simulink model "car_speed_control_simulation2"  (R2024b)
settings: Solver=VariableStepAuto  StartTime=0.0  StopTime=500  RelTol=1e-3
libraries: simulink_extras x2
settings Model: Creator=USER  LastModifiedBy=USER

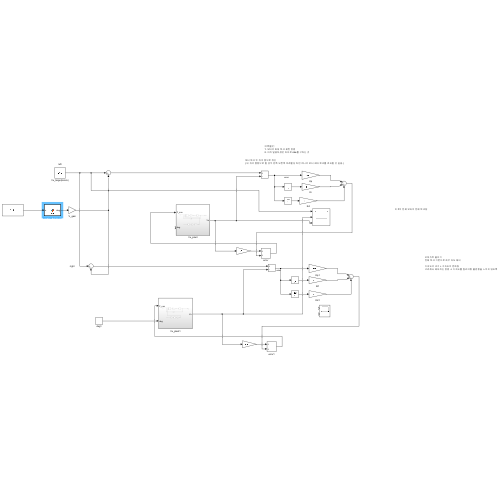
[thumbnail: Simulink's stored preview of the top-level diagram]
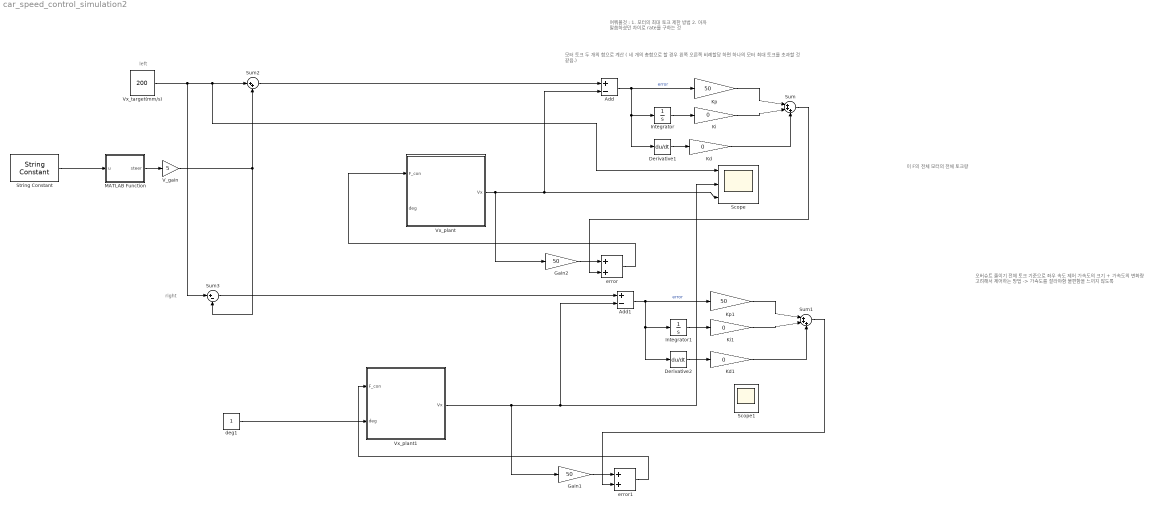
== system car_speed_control_simulation2 ==
  note: left
  note: 여쭤볼것 :
      | 1. 모터의 최대 토크 제한 방법
      | 2. 아까 말씀하셨던 차이로 rate를 구하는 것
  note: 모터 토크 두 개의 합으로 계산
      | ( 네 개의 총합으로 할 경우 왼쪽 오른쪽 비례할당 하면 하나의 모터 최대 토크를 초과할 것 같음.)
  note: 이 F의 전체 모터의 전체 토크량
  note: 오버슈트 줄이기
      | 전체 토크 기준으로 좌우 속도 제어
      |
      | 가속도의 크기 + 가속도의 변화량
      | 고려해서 제어하는 방법 -> 가속도를 잘라야함 불편함을 느끼지 않도록
  note: right
  Add : Sum  Inputs=+-
  Add1 : Sum  Inputs=+-
  Derivative1 : Derivative
  Derivative2 : Derivative
  Gain1 : Gain  Gain=50
  Gain2 : Gain  Gain=50
  Integrator : Integrator
  Integrator1 : Integrator
  Kd : Gain  Gain=0
  Kd1 : Gain  Gain=0
  Ki : Gain  Gain=0
  Ki1 : Gain  Gain=0
  Kp : Gain  Gain=50
  Kp1 : Gain  Gain=50
  MATLAB Function : MATLAB Function  TreatAsAtomicUnit=on
  Scope : Scope  NumInputPorts=3
  Scope1 : Scope  NumInputPorts=2
  String Constant : StringConstant  String="\"1,0\""
  Sum : Sum  Inputs=|+++
  Sum1 : Sum  Inputs=|+++
  Sum2 : Sum  Inputs=|++
  Sum3 : Sum  Inputs=|+-
  V_gain : Gain  Gain=5
  Vx_plant : Subsystem
  Vx_plant1 : Subsystem
  Vx_target(mm/s) : Constant  Value=200
  deg1 : Constant
  error : Sum
  error1 : Sum
  wires:
  Vx_plant/1(Vx) -> Add/2, Scope/3, Gain2/1
  Add/1 -> Derivative1/1, Integrator/1, Kp/1  "error"
  Gain2/1 -> error/1
  error/1 -> Vx_plant/1(F_con)
  MATLAB Function/1(steer) -> V_gain/1
  Integrator/1 -> Ki/1
  Derivative1/1 -> Kd/1
  Kp/1 -> Sum/1
  Ki/1 -> Sum/2
  Kd/1 -> Sum/3
  Sum/1 -> error/2
  Sum1/1 -> error1/2
  Kd1/1 -> Sum1/3
  Ki1/1 -> Sum1/2
  Kp1/1 -> Sum1/1
  Derivative2/1 -> Kd1/1
  Integrator1/1 -> Ki1/1
  deg1/1 -> Vx_plant1/2(deg)
  error1/1 -> Vx_plant1/1(F_con)
  Gain1/1 -> error1/1
  Vx_plant1/1(Vx) -> Gain1/1, Scope/2, Add1/2
  Vx_target(mm/s)/1 -> Sum3/1, Scope/1, Sum2/1
  Sum2/1 -> Add/1
  String Constant/1 -> MATLAB Function/1(u)
  V_gain/1 -> Sum2/2, Sum3/2
  Sum3/1 -> Add1/1
  Add1/1 -> Integrator1/1, Derivative2/1, Kp1/1  "error"

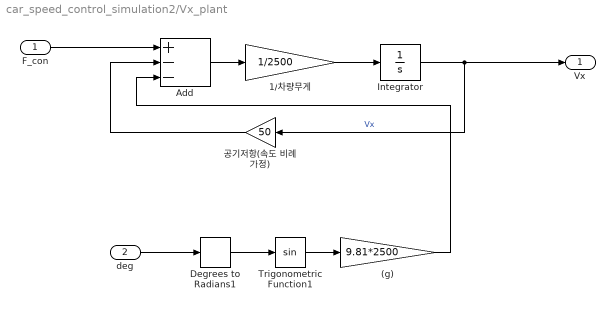
== system car_speed_control_simulation2/Vx_plant ==
  F_con : Inport
  deg : Inport  Port=2
  (g) : Gain  Gain=9.81*2500
  1/차량무게 : Gain  Gain=1/2500
  Add : Sum  Inputs=+--
  Degrees to Radians1 : simulink_extras/Transformations/Degrees to Radians
  Integrator : Integrator
  Trigonometric Function1 : Trigonometry
  공기저항(속도 비례 가정) : Gain  Gain=50
  Vx : Outport
  wires:
  Integrator/1 -> Vx/1, 공기저항(속도 비례 가정)/1  "Vx"
  Add/1 -> 1/차량무게/1
  F_con/1 -> Add/1
  1/차량무게/1 -> Integrator/1
  공기저항(속도 비례 가정)/1 -> Add/2
  Degrees to Radians1/1 -> Trigonometric Function1/1
  Trigonometric Function1/1 -> (g)/1
  deg/1 -> Degrees to Radians1/1
  (g)/1 -> Add/3

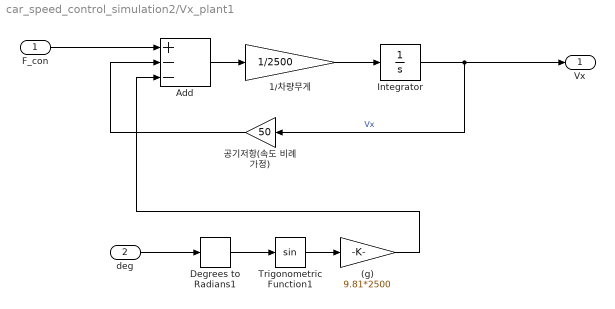
== system car_speed_control_simulation2/Vx_plant1 ==
  F_con : Inport
  deg : Inport  Port=2
  (g) : Gain  Gain=9.81*2500
  1/차량무게 : Gain  Gain=1/2500
  Add : Sum  Inputs=+--
  Degrees to Radians1 : simulink_extras/Transformations/Degrees to Radians
  Integrator : Integrator
  Trigonometric Function1 : Trigonometry
  공기저항(속도 비례 가정) : Gain  Gain=50
  Vx : Outport
  wires:
  (g)/1 -> Add/3
  deg/1 -> Degrees to Radians1/1
  Trigonometric Function1/1 -> (g)/1
  Degrees to Radians1/1 -> Trigonometric Function1/1
  공기저항(속도 비례 가정)/1 -> Add/2
  1/차량무게/1 -> Integrator/1
  F_con/1 -> Add/1
  Add/1 -> 1/차량무게/1
  Integrator/1 -> 공기저항(속도 비례 가정)/1, Vx/1  "Vx"

== matlab function car_speed_control_simulation2/MATLAB Function ==
  data: u input; steer output
function steer = fcn(u)
    str = char(u);
    neg_flag = 0;
    steer= 0;
    
    idxs = find(str == ',');
    if length(idxs) >= 1
        idx1 = idxs(1);
        
        s1 = str(1:idx1-1);
        s2 = str(idx1+1:end);
       
        neg_flag = real(str2double(s1));
        steer   = real(str2double(s2));
    end

    if(neg_flag==1)
        steer = steer * -1;
    end
